simulink model "untitled1"  (R2020b)
settings: Solver=VariableStepAuto  StartTime=0.0  StopTime=1.0  RelTol=1e-3
values from neighbouring files (symbols this model uses):
  A = [0 1 0 0 ... (first row only)    [state_space_vars.m]
  B = [0; B1; 0; B3]    [state_space_vars.m]
  C = [0 0 1 0]    [state_space_vars.m]
  D = [0]    [state_space_vars.m]
  x0 = [0; 0; -3*pi/180; 0]    [compare_models.m]
settings Model: Creator=olivergrainge  LastModifiedBy=olivergrainge

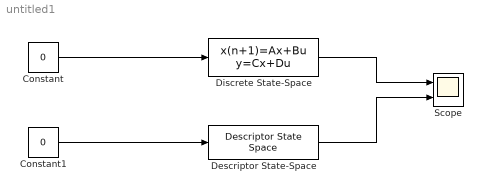
== system untitled1 ==
  Constant : Constant  Value=0
  Constant1 : Constant  Value=0
  Descriptor State-Space : DescriptorStateSpace  E=ones(4)  A=A  B=B  C=C  D=D  InitialCondition=x0
  Discrete State-Space : DiscreteStateSpace  A=A  B=B  C=C  D=D  InitialCondition=x0  SampleTime=-1
  Scope : Scope  NumInputPorts=2
  wires:
  Constant/1 -> Discrete State-Space/1
  Constant1/1 -> Descriptor State-Space/1
  Descriptor State-Space/1 -> Scope/2
  Discrete State-Space/1 -> Scope/1
